simulink model "calcThrTension_th"  (R2020a)
settings: Solver=VariableStepAuto  StartTime=0.0  StopTime=1  RelTol=1e-3
libraries: calcThrTension_ul x1
settings Model: Creator=Ayaz  LastModifiedBy=Ayaz

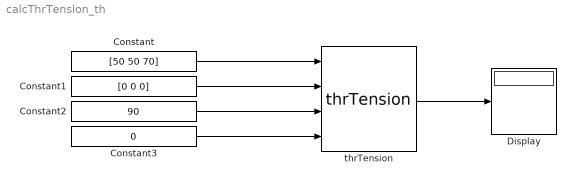
== system calcThrTension_th ==
  Constant : Constant  Value=[50 50 70]
  Constant1 : Constant  Value=[0 0 0]
  Constant2 : Constant  Value=90
  Constant3 : Constant  Value=0
  Display : Display
  thrTension : calcThrTension_ul/thrTension  thrSpringCns=100
  wires:
  Constant/1 -> thrTension/1
  Constant1/1 -> thrTension/2
  Constant2/1 -> thrTension/3
  Constant3/1 -> thrTension/4
  thrTension/1 -> Display/1
